simulink model "LKA"  (R2021a)
settings: Solver=FixedStepAuto  StartTime=0.0  StopTime=43  FixedStep=0.05  MaxStep=0.05  RelTol=1e3
undefined symbols (not defined in the file or in its folder): car, curvatures, directions, refPoses, speedProfile, Ts
libraries: simulink_extras x2, pid_lib x1, drivingscenarioandsensors x1, car_library x1
settings Model: Creator=efrem  LastModifiedBy=efrem
settings SolverCC: SolverResetMethod=Robust

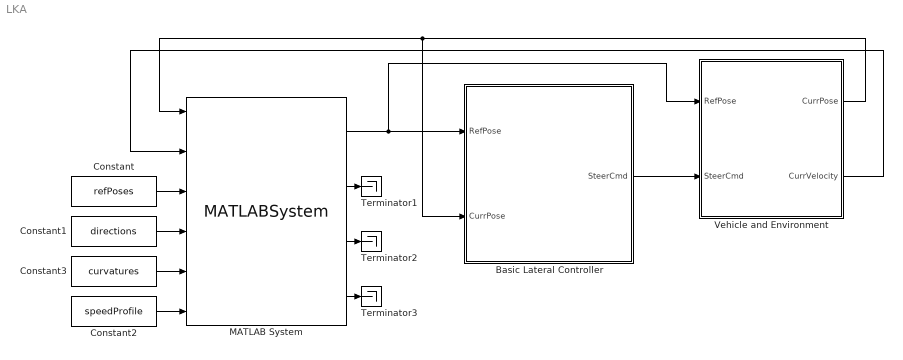
== system LKA ==
  Basic Lateral Controller : Subsystem
  Constant : Constant  Value=refPoses
  Constant1 : Constant  Value=directions
  Constant2 : Constant  Value=speedProfile
  Constant3 : Constant  Value=curvatures
  MATLAB System : MATLABSystem  System=HelperPathAnalyzer  Wheelbase=2.8  HasResetOutput=off  SimulateUsing=Interpreted execution
      mask Type: HelperPathAnalyzer
      mask Display:
      | disp(['Helper' char(10) 'Path' char(10) 'Analyzer']);
      | port_label('input',1,'CurrPose');
      | port_label('input',2,'CurrVelocity');
      | port_label('input',3,'RefPoses');
      | port_label('input',4,'Directions');
      | port_label('input',5,'Curvatures');
      | port_label('input',6,'RefVelocities');
      | port_label('output',1,'RefPose');
      | port_label('output',2,'RefVelocity');
      | port_label('output',3,'Direction');
      | port_label('output',4,'Curvature');
  Terminator1 : Terminator
  Terminator2 : Terminator
  Terminator3 : Terminator
  Vehicle and Environment : Subsystem
  wires:
  MATLAB System/3 -> Terminator2/1
  MATLAB System/4 -> Terminator3/1
  Vehicle and Environment/2(CurrVelocity) -> MATLAB System/2
  Vehicle and Environment/1(CurrPose) -> Basic Lateral Controller/2(CurrPose), MATLAB System/1
  Constant/1 -> MATLAB System/3
  Constant2/1 -> MATLAB System/6
  Basic Lateral Controller/1(SteerCmd) -> Vehicle and Environment/2(SteerCmd)
  MATLAB System/2 -> Terminator1/1
  Constant3/1 -> MATLAB System/5
  MATLAB System/1 -> Vehicle and Environment/1(RefPose), Basic Lateral Controller/1(RefPose)
  Constant1/1 -> MATLAB System/4

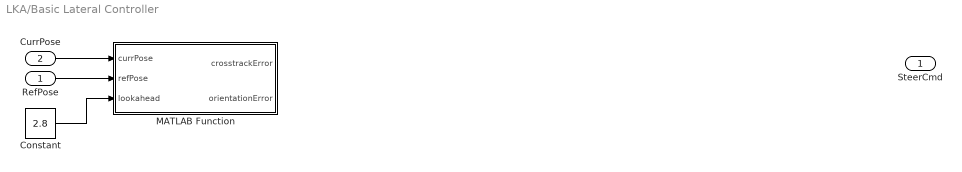
== system LKA/Basic Lateral Controller ==
  RefPose : Inport
  CurrPose : Inport  Port=2
  Constant : Constant  Value=2.8
  MATLAB Function : MATLAB Function  TreatAsAtomicUnit=on
  SteerCmd : Outport
  wires:
  CurrPose/1 -> MATLAB Function/1(currPose)
  RefPose/1 -> MATLAB Function/2(refPose)
  Constant/1 -> MATLAB Function/3(lookahead)

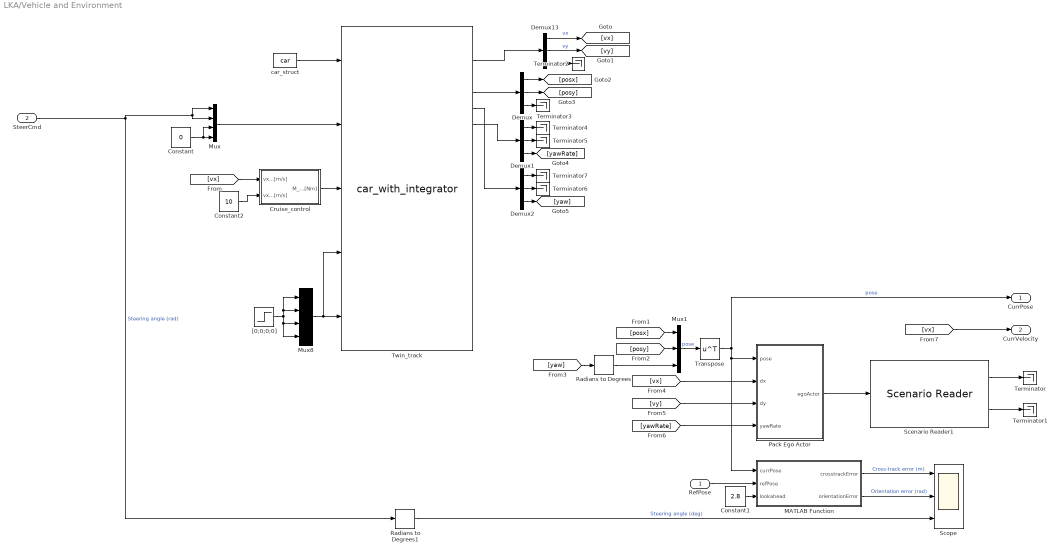
== system LKA/Vehicle and Environment ==
  RefPose : Inport
  SteerCmd : Inport  Port=2
  Constant : Constant  Value=0
  Constant1 : Constant  Value=2.8
  Constant2 : Constant  Value=10
  Cruise_control : Subsystem
  Demux{,1..2,13} (4 alike) : Demux  Outputs=3
  MATLAB Function : MATLAB Function  TreatAsAtomicUnit=on
  Mux : Mux
  Mux1 : Mux  Inputs=3
  Mux8 : Mux
  Pack Ego Actor : MATLAB Function  TreatAsAtomicUnit=on
  Radians to Degrees : simulink_extras/Transformations/Radians to Degrees
  Radians to Degrees1 : simulink_extras/Transformations/Radians to Degrees
  Scenario Reader1 : drivingscenarioandsensors/Scenario Reader  ScenarioSource=From file  ScenarioFileName=LateralControl.mat  ScenarioVariableName=scenario  OutputCoordinateSystem=Vehicle coordinates  EgoVehicleSource=Input port  EgoVehicleActorID=1  OrientVehiclesOnRoad=off  OutputEgoVehiclePose=off  SampleTime=Ts  LaneBoundaryOutput=Ego vehicle lane boundaries  LaneBoundaryDistance=0:0.5:9.5  LaneBoundaryLocation=Center of lane markings  BusNameSource=Property  BusName=BusActors  BusNumActorsSource=Scenario  BusNumActors=100  BusName2Source=Auto  BusName2=BusLaneBoundaries  BusNumLaneBoundariesSource=Scenario  BusNumLaneBoundaries=10  BusName3Source=Auto  BusName3=BusEgoActor  ShowCoordinateLabels=on  SimulateUsing=Interpreted execution
  Scope : Scope  NumInputPorts=3
  Terminator{,1..7} (8 alike) : Terminator
  Transpose : Math  Operator=transpose  SignedPower=on  SaturateOnIntegerOverflow=on
  Twin_track : car_library/car_with_integrator  SystemSampleTime=-1  VariantActivationTime=update diagram  Latency=0  AutoFrameSizeCalculation=off
  "[0;0;0;0]" : Step  Time=0  After=0  SampleTime=0
  car_struct : Constant  Value=car  OutDataTypeStr=Bus: car_bus
  CurrPose : Outport  VectorParamsAs1DForOutWhenUnconnected=off
  CurrVelocity : Outport  Port=2  VectorParamsAs1DForOutWhenUnconnected=off
  wires:
  [vx] -> Pack Ego Actor/2(dx)
  [yawRate] -> Pack Ego Actor/4(yawRate)
  [vy] -> Pack Ego Actor/3(dy)
  Transpose/1 -> CurrPose/1, MATLAB Function/1(currPose), Pack Ego Actor/1(pose)  "pose"
  MATLAB Function/1(crosstrackError) -> Scope/1  "Cross-track error (m)"
  RefPose/1 -> MATLAB Function/2(refPose)
  MATLAB Function/2(orientationError) -> Scope/2  "Orientation error (rad)"
  Scenario Reader1/1 -> Terminator/1
  [vx] -> CurrVelocity/1
  Scenario Reader1/2 -> Terminator1/1
  Pack Ego Actor/1(egoActor) -> Scenario Reader1/1
  SteerCmd/1 -> Mux/1, Mux/2, Radians to Degrees1/1  "Steering angle (rad)"
  Constant1/1 -> MATLAB Function/3(lookahead)
  Mux8/1 -> Twin_track/4, Twin_track/5
  Cruise_control/1(M_m_d [Nm]) -> Twin_track/3
  car_struct/1 -> Twin_track/1
  "[0;0;0;0]"/1 -> Mux8/2, Mux8/1, Mux8/4, Mux8/3
  Demux13/3 -> Terminator2/1
  Twin_track/2 -> Demux13/1
  Demux13/2 -> [vy]  "vy"
  Constant2/1 -> Cruise_control/2(vx_ref [m/s])
  Constant/1 -> Mux/3, Mux/4
  Mux/1 -> Twin_track/2
  Twin_track/4 -> Demux/1
  Demux13/1 -> [vx]  "vx"
  [vx] -> Cruise_control/1(vx_twin [m/s])
  Demux/1 -> [posx]
  Demux/2 -> [posy]
  Demux/3 -> Terminator3/1
  Twin_track/6 -> Demux1/1
  Demux1/1 -> Terminator4/1
  Demux1/2 -> Terminator5/1
  Demux1/3 -> [yawRate]
  Twin_track/5 -> Demux2/1
  Demux2/3 -> [yaw]
  Demux2/2 -> Terminator6/1
  Demux2/1 -> Terminator7/1
  [posx] -> Mux1/1
  [posy] -> Mux1/2
  Radians to Degrees/1 -> Mux1/3
  Mux1/1 -> Transpose/1  "pose"
  [yaw] -> Radians to Degrees/1
  Radians to Degrees1/1 -> Scope/3  "Steering angle (deg)"

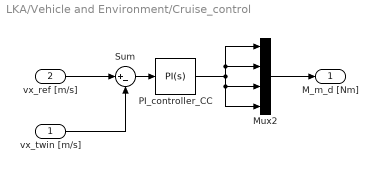
== system LKA/Vehicle and Environment/Cruise_control ==
  vx_twin [m/s] : Inport
  vx_ref [m/s] : Inport  Port=2
  Mux2 : Mux
  PI_controller_CC : pid_lib/PID Controller  Controller=PI  Form=Parallel  TimeDomain=Continuous-time  UseExternalTs=off  SampleTime=-1  IntegratorMethod=Forward Euler  FilterMethod=Forward Euler  ControllerParametersSource=internal  P=100  I=100  D=0  UseFilter=on  N=100  TunerSelectOption=Transfer Function Based (PID Tuner App)  InitialConditionSource=internal  InitialConditionForIntegrator=0  InitialConditionForFilter=0  DifferentiatorICPrevScaledInput=0  ExternalReset=none  TrackingMode=off  Kt=1  LimitOutput=on  SatLimitsSource=internal  UpperSaturationLimit=inf  LowerSaturationLimit=0  LinearizeAsGain=on  AntiWindupMode=clamping  Kb=1  POutMin=[]  POutMax=[]  IOutMin=[]  IOutMax=[]  DOutMin=[]  DOutMax=[]  NOutMin=[]  NOutMax=[]  SumOutMin=[]  SumOutMax=[]  SaturationOutMin=[]  SaturationOutMax=[]  PParamMin=[]  PParamMax=[]  IParamMin=[]  IParamMax=[]  DParamMin=[]  DParamMax=[]  NParamMin=[]  NParamMax=[]  KbParamMin=[]  KbParamMax=[]  KtParamMin=[]  KtParamMax=[]  KbOutMin=[]  KbOutMax=[]  KtOutMin=[]  KtOutMax=[]  IntegratorOutMin=[]  IntegratorOutMax=[]  FilterOutMin=[]  FilterOutMax=[]  SumI1OutMin=[]  SumI1OutMax=[]  SumI2OutMin=[]  SumI2OutMax=[]  SumI3OutMin=[]  SumI3OutMax=[]  SumI4OutMin=[]  SumI4OutMax=[]  SumDOutMin=[]  SumDOutMax=[]  DifferentiatorOutMin=[]  DifferentiatorOutMax=[]  FilterDiffOutCoefMin=[]  FilterDiffOutCoefMax=[]  ReciprocalOutMin=[]  ReciprocalOutMax=[]  SumDenOutMin=[]  SumDenOutMax=[]  SumNumOutMin=[]  SumNumOutMax=[]  DivideOutMin=[]  DivideOutMax=[]  UdiffTsProdOutMin=[]  UdiffTsProdOutMax=[]  NTsProdOutMin=[]  NTsProdOutMax=[]  UintegralTsProdOutMin=[]  UintegralTsProdOutMax=[]  UngainTsProdOutMin=[]  UngainTsProdOutMax=[]  IntegratorContinuousStateAttributes=''  IntegratorStateMustResolveToSignalObject=off  IntegratorRTWStateStorageClass=Auto  FilterContinuousStateAttributes=''  FilterStateMustResolveToSignalObject=off  FilterRTWStateStorageClass=Auto  ParallelPVariant=InternalParameters  IdealPVariant=Disabled  IVariant=InternalParameters  DVariant=Disabled  IntegratorVariant=Continuous  SatVariant=Enabled  AWVariant=ContClampingParallel  PCopyVariant=Disabled  TRVariant=Disabled  FdbkBlocksVariant=Forward  IdealPFdbkVariant=Disabled  SatFdbkVariant=Disabled  DerivativeFilterVariant=Disabled  NVariant=Disabled  NCopyVariant=Disabled_SignalSpec  FilterICVariant=Disabled  IntegratorICVariant=InternalICs  ExternalResetVariant=Disabled  TRSumVariant=Passthrough  SumFdbkVariant=Disabled  SumVariant=Sum_PI  TsampFilterVariant=InternalTs  TsampNgainVariant=Passthrough  TsampIntegralVariant=Passthrough  ExternalSaturationOutDataTypeStr=Inherit: Same as second input
  Sum : Sum  Inputs=|+-
  M_m_d [Nm] : Outport
  wires:
  vx_ref [m/s]/1 -> Sum/1
  vx_twin [m/s]/1 -> Sum/2
  Sum/1 -> PI_controller_CC/1
  Mux2/1 -> M_m_d [Nm]/1
  PI_controller_CC/1 -> Mux2/4, Mux2/3, Mux2/2, Mux2/1

== matlab function LKA/Vehicle and Environment/MATLAB Function ==
  data: currPose input; crosstrackError output; refPose input; lookahead input; orientationError output
function [crosstrackError, orientationError] = fcn(currPose, refPose, lookahead)

currPose(3) = deg2rad(currPose(3));
refPose(3) = deg2rad(refPose(3));

currPoseFollowedPoint = zeros(1,2);
currPoseFollowedPoint(1) = currPose(1) + lookahead * cos(currPose(3));
currPoseFollowedPoint(2) = currPose(2) + lookahead * sin(currPose(3));

crosstrackError = sign(refPose(2) - currPoseFollowedPoint(2))*...
    norm(currPoseFollowedPoint(1:2) - refPose(1:2));

orientationError = currPose(3) - refPose(3);

== matlab function LKA/Basic Lateral Controller/MATLAB Function ==
  data: currPose input; crosstrackError output; refPose input; lookahead input; orientationError output
function [crosstrackError, orientationError] = fcn(currPose, refPose, lookahead)

currPose(3) = deg2rad(currPose(3));
refPose(3) = deg2rad(refPose(3));

currPoseFollowedPoint = zeros(1,2);
currPoseFollowedPoint(1) = currPose(1) + lookahead * cos(currPose(3));
currPoseFollowedPoint(2) = currPose(2) + lookahead * sin(currPose(3));

crosstrackError = sign(refPose(2) - currPoseFollowedPoint(2))*...
    norm(currPoseFollowedPoint(1:2) - refPose(1:2));

orientationError = currPose(3) - refPose(3);

== matlab function LKA/Vehicle and Environment/Pack Ego Actor ==
  data: pose input; egoActor output Bus: BusActorsActors size=1; dx input; dy input; yawRate input
function egoActor = packEgo(pose,dx,dy,yawRate)
% Pack ego information into a single ego actor bus
%
% Imoprtant note:
% Output is a bus of type BusActorsActors. This is the same bus used by the
% Scenario Reader to output an individual actor. If you change the
% output bus name of Scenario Reader, change the output bus name here
% as well by clicking on 'Edit Data' in the menu above.

egoActor = struct(...
    'ActorID', 1,...
    'Position', [pose(1) pose(2) 0], ...
    'Velocity', [dx dy 0], ...
    'Roll', 0, ...
    'Pitch', 0, ...
    'Yaw', pose(3), ...
    'AngularVelocity', [0 0 yawRate]);
